simulink library "powerlib_modelsV2"  (Simulink 6.0)
settings: Solver=ode45  SolverMode=SingleTasking  StartTime=0.0  StopTime=10.0  RelTol=1e-3
values from neighbouring files (symbols this model uses):
  Ts = get(handles.edit1,'string')    [powergui.m]
undefined symbols (not defined in the file or in its folder): A, Ac, B, Bc, C, Cc, Cs, Current, damp, Dc, Dd, DiscIntNeverNeededParam, dref, dwo, exc, F, fb, gate, GH, GHd, GI, GId, GL, GLd, H, HT, hyd, ib, ib2, io, isfinite, j, K, Kd, Kg, L, Lad, Laq, lim, LIM, Ll, Llfd, Llkd, Llkq1, Llkq2, Llr, Lls, LowerFlux, N, N2, Nb, Nb2, nb_arm, p, Par_HarmoA_pu, Par_HarmoB_pu, Par_Timing_Harmo, Par_Timing_Variation, Par_Vps, Pb ... (+57)
libraries: powerlib_extras x14
(part 9 of 11)

== system powerlib_modelsV2/Discrete/synchronous_machine/phiq ==
  note: This subsystem computes the quadrature axis flux phiq.
  vq : Inport  Port=1  LatchInput=off
  w : Inport  Port=2  LatchInput=off
  phid : Inport  Port=3  LatchInput=off
  phimq : Inport  Port=4  LatchInput=off
  Discrete-Time Integrator : DiscreteIntegrator  IntegratorMethod=Integration: Trapezoidal  InitialCondition=phiqo  SampleTime=Ts  SaturateOnIntegerOverflow=on  ICPrevOutput=DiscIntNeverNeededParam  ICPrevScaledInput=DiscIntNeverNeededParam
  Product2 : Product  SaturateOnIntegerOverflow=on  InputSameDT=on
  Rs_Ll : Gain  Gain=Rs/Ll  SaturateOnIntegerOverflow=on
  Sum : Sum  Inputs=+-+  SaturateOnIntegerOverflow=on  InputSameDT=on
  Sum6 : Sum  Inputs=+-  SaturateOnIntegerOverflow=on  InputSameDT=on
  Unit Delay1 : UnitDelay  X0=phiqo  SampleTime=Ts
  web_psb : Gain  Gain=web_psb  SaturateOnIntegerOverflow=on
  phiq : Outport  InitialOutput=0
  wires:
  Discrete-Time Integrator/1 -> Unit Delay1/1
  web_psb/1 -> Discrete-Time Integrator/1
  phimq/1 -> Sum6/1
  phid/1 -> Product2/2
  w/1 -> Product2/1
  vq/1 -> Sum/1
  Product2/1 -> Sum/2
  Sum6/1 -> Rs_Ll/1
  Rs_Ll/1 -> Sum/3
  Sum/1 -> web_psb/1
  Unit Delay1/1 -> phiq/1, Sum6/2

== system powerlib_modelsV2/Discrete/synchronous_machine/qd2abc ==
  note: This subsystem converts id,iq to ia,ib,ic.
  sin,cos : Inport  Port=1  LatchInput=off
  iq,id : Inport  Port=2  LatchInput=off
  Fcn : Fcn  Expr=u[3]*u[2] + u[4]*u[1]
  Fcn1 : Fcn  Expr=(u[2]*(-u[3]-sqrt3*u[4]) + u[1]*(sqrt3*u[3]-u[4]))*0.5
  Mux : Mux  Inputs=[ 2 2 ]
  Mux1_ : Mux  Inputs=3
  Sum : Sum  Orientation=down  Inputs=--  SaturateOnIntegerOverflow=on  InputSameDT=on
  ib : Gain  Gain=ib  SaturateOnIntegerOverflow=on
  is(A) : Outport  InitialOutput=0
  is(pu) : Outport  Port=2  InitialOutput=0
  wires:
  ib/1 -> is(A)/1
  Fcn1/1 -> Sum/2, Mux1_/2
  Fcn/1 -> Mux1_/1, Sum/1
  Sum/1 -> Mux1_/3
  Mux1_/1 -> ib/1, is(pu)/1
  Mux/1 -> Fcn/1, Fcn1/1
  sin,cos/1 -> Mux/1
  iq,id/1 -> Mux/2

== system powerlib_modelsV2/Phasors/3_Phase_Prog_Source/Seq A Generation ==
  Enable : Inport  Port=1  LatchInput=off
  Gain3 : Gain  Gain=pi/180  SaturateOnIntegerOverflow=on
  Magnitude-Angle to Complex : MagnitudeAngleToComplex
  Multiport Switch : MultiPortSwitch  Inputs=3  InputSameDT=on
  Negative-sequence : Constant  Value=[0 2*pi/3 -2*pi/3]
  Phase_Harmo : Constant  Value=Phase_Harmo
  Phase_Harmo1 : Constant  Value=Mag_Harmo
  Phase_Harmo2 : Constant  Value=Seq_Harmo
  Positive-sequence : Constant  Value=[0 -2*pi/3 2*pi/3]
  Product1 : Product  SaturateOnIntegerOverflow=on  InputSameDT=on
  Sum : Sum  SaturateOnIntegerOverflow=on  InputSameDT=on
  Sum1 : Sum  SaturateOnIntegerOverflow=on  InputSameDT=on
  Zero-sequence : Constant  Value=[0 0 0]
  valp_nom2 : Constant
  Seq120 : Outport
  wires:
  Enable/1 -> Product1/1
  Phase_Harmo1/1 -> Magnitude-Angle to Complex/1
  Multiport Switch/1 -> Sum/2
  Phase_Harmo/1 -> Gain3/1
  valp_nom2/1 -> Sum1/2
  Phase_Harmo2/1 -> Sum1/1
  Sum1/1 -> Multiport Switch/1
  Product1/1 -> Seq120/1
  Magnitude-Angle to Complex/1 -> Product1/2
  Gain3/1 -> Sum/1
  Negative-sequence/1 -> Multiport Switch/4
  Positive-sequence/1 -> Multiport Switch/3
  Zero-sequence/1 -> Multiport Switch/2
  Sum/1 -> Magnitude-Angle to Complex/2

== system powerlib_modelsV2/Phasors/3_Phase_Prog_Source/Seq B Generation ==
  Enable : Inport  Port=1  LatchInput=off
  Gain3 : Gain  Gain=pi/180  SaturateOnIntegerOverflow=on
  Magnitude-Angle to Complex : MagnitudeAngleToComplex
  Multiport Switch : MultiPortSwitch  Inputs=3  InputSameDT=on
  Negative-sequence : Constant  Value=[0 2*pi/3 -2*pi/3]
  Phase_Harmo : Constant  Value=Phase_Harmo
  Phase_Harmo1 : Constant  Value=Mag_Harmo
  Phase_Harmo2 : Constant  Value=Seq_Harmo
  Positive-sequence : Constant  Value=[0 -2*pi/3 2*pi/3]
  Product1 : Product  SaturateOnIntegerOverflow=on  InputSameDT=on
  Sum : Sum  SaturateOnIntegerOverflow=on  InputSameDT=on
  Sum1 : Sum  SaturateOnIntegerOverflow=on  InputSameDT=on
  Zero-sequence : Constant  Value=[0 0 0]
  valp_nom2 : Constant
  Seq120 : Outport
  wires:
  Sum/1 -> Magnitude-Angle to Complex/2
  Zero-sequence/1 -> Multiport Switch/2
  Positive-sequence/1 -> Multiport Switch/3
  Negative-sequence/1 -> Multiport Switch/4
  Gain3/1 -> Sum/1
  Magnitude-Angle to Complex/1 -> Product1/2
  Product1/1 -> Seq120/1
  Sum1/1 -> Multiport Switch/1
  Phase_Harmo2/1 -> Sum1/1
  valp_nom2/1 -> Sum1/2
  Phase_Harmo/1 -> Gain3/1
  Multiport Switch/1 -> Sum/2
  Phase_Harmo1/1 -> Magnitude-Angle to Complex/1
  Enable/1 -> Product1/1

== system powerlib_modelsV2/Phasors/3_Phase_Prog_Source/Timer ==
  Clock : Clock
  Look-Up Table : Lookup  DialogController=Simulink.DDGSource  InputValues=tv  OutputValues=opv  SaturateOnIntegerOverflow=on
  Out : Outport
  wires:
  Clock/1 -> Look-Up Table/1
  Look-Up Table/1 -> Out/1

== system powerlib_modelsV2/Phasors/3_Phase_Prog_Source/Variation SubSystem ==
  VariationType : Inport  Port=1  LatchInput=off
  Constant : Constant  Value=2
  Constant1 : Constant  Value=0
  Constant2 : Constant
  Constant3 : Constant
  Constant4 : Constant  Value=0
  Constant5 : Constant  Value=0
  Data Type  Conversion1 : DataTypeConversion  SaturateOnIntegerOverflow=on  RndMeth=Zero
  Data Type  Conversion2 : DataTypeConversion  Orientation=up  SaturateOnIntegerOverflow=on  RndMeth=Zero
  Gain1 : Gain  Gain=2*pi  SaturateOnIntegerOverflow=on
  Integrator : Integrator
  Logical Operator : Logic
  Logical Operator1 : Logic  Orientation=up  Operator=NOT
  Memory : Memory  Orientation=left
  Multiport Switch1 : MultiPortSwitch  InputSameDT=on
  Product : Product  SaturateOnIntegerOverflow=on  InputSameDT=on
  Product1 : Product  SaturateOnIntegerOverflow=on  InputSameDT=on
  Product2 : Product  SaturateOnIntegerOverflow=on  InputSameDT=on
  Relational Operator : RelationalOperator  Operator===  InputSameDT=on
  Relational Operator1 : RelationalOperator  Operator===  InputSameDT=on
  Step : Step  Time=Ton_Variation  SampleTime=0
  Step1 : Step  Time=Toff_Variation  Before=1  After=0  SampleTime=0
  Switch{,1..3} (4 alike) : Switch  Threshold=0.5  InputSameDT=on
  Trigonometric Function1 : Trigonometry
  valp_nom6 : Constant  Value=VariationStep
  valp_nom7 : Constant  Value=VariationRate
  valp_nom8 : Constant  Value=VariationMag
  valp_nom9 : Constant  Value=VariationFreq
  Value : Outport
  wires:
  Relational Operator1/1 -> Data Type  Conversion1/1
  Data Type  Conversion2/1 -> Logical Operator1/1
  Trigonometric Function1/1 -> Product/2
  valp_nom8/1 -> Product/1
  valp_nom9/1 -> Gain1/1
  Gain1/1 -> Product1/2
  Product1/1 -> Trigonometric Function1/1
  Product/1 -> Multiport Switch1/4  "Mod"
  valp_nom7/1 -> Switch1/1
  Constant2/1 -> Switch1/3
  Constant4/1 -> Switch/3
  Switch1/1 -> Switch/1
  Constant/1 -> Relational Operator/2
  Switch/1 -> Integrator/1
  Relational Operator/1 -> Switch1/2
  valp_nom6/1 -> Product2/1
  Product2/1 -> Multiport Switch1/2  "Step"
  Integrator/1 -> Product1/1, Multiport Switch1/3  "Ramp"
  VariationType/1 -> Multiport Switch1/1, Relational Operator1/1, Relational Operator/1
  Step/1 -> Switch/2, Product2/2  "Ton"
  Multiport Switch1/1 -> Switch2/1
  Memory/1 -> Switch2/3
  Constant1/1 -> Switch3/1
  Switch2/1 -> Memory/1, Switch3/3
  Switch3/1 -> Value/1
  Constant3/1 -> Relational Operator1/2
  Step1/1 -> Data Type  Conversion2/1, Switch2/2  "Toff"
  Logical Operator/1 -> Switch3/2
  Logical Operator1/1 -> Logical Operator/1
  Constant5/1 -> Multiport Switch1/5
  Data Type  Conversion1/1 -> Logical Operator/2

== system powerlib_modelsV2/Phasors/Dynamic_Load/Break  Alg. Loop I1 ==
  In : Inport  Orientation=left  Port=1  LatchInput=off
  Complex to Real-Imag : ComplexToRealImag  Orientation=left
  Real-Imag to Complex : RealImagToComplex  Orientation=left
  imag : Subsystem  Orientation=left  mask(Transfer Function with Initial Outputs){N=[1], D=[100e-6  1], Y0=imag(I1_init), U0=imag(I1_init)}
      mask prompts: N "Numerator:"; D "Denominator:"; Y0 "Initial output:"; U0 "Initial input:"
      mask help: Vector expressions for numerator, and denominator. Coefficients are in descending powers of s.
      mask init:
      | [A,B,C,Dd]=tf2ss(N,D);if (isempty(Y0));[m,n]=size(A);X0=zeros(1,m); end; if (isempty(U0));[m,p]=size(B);U0=zeros(1,p);end;X0=getxo(A,B,C,Dd,U0,Y0,0);
      mask Help: Specify the initial output for the transfer function.  An optimization routine attempts to determine the appropriate initial states so that the specified initial output is achieved.  For more details, see the m-file getxo.m
      mask Display: dpoly(N,D,'s')
  real : Subsystem  Orientation=left  mask(Transfer Function with Initial Outputs){N=[1], D=[100e-6  1], Y0=real(I1_init), U0=real(I1_init)}
      mask prompts: N "Numerator:"; D "Denominator:"; Y0 "Initial output:"; U0 "Initial input:"
      mask help: Vector expressions for numerator, and denominator. Coefficients are in descending powers of s.
      mask init:
      | [A,B,C,Dd]=tf2ss(N,D);if (isempty(Y0));[m,n]=size(A);X0=zeros(1,m); end; if (isempty(U0));[m,p]=size(B);U0=zeros(1,p);end;X0=getxo(A,B,C,Dd,U0,Y0,0);
      mask Help: Specify the initial output for the transfer function.  An optimization routine attempts to determine the appropriate initial states so that the specified initial output is achieved.  For more details, see the m-file getxo.m
      mask Display: dpoly(N,D,'s')
  Out : Outport  Orientation=left
  wires:
  imag/1(Out1) -> Real-Imag to Complex/2
  Complex to Real-Imag/2 -> imag/1(In1)
  real/1(Out1) -> Real-Imag to Complex/1
  Complex to Real-Imag/1 -> real/1(In1)
  Real-Imag to Complex/1 -> Out/1
  In/1 -> Complex to Real-Imag/1

== system powerlib_modelsV2/Phasors/Dynamic_Load/I1  ==
  note: V2= 1/3(Vab -a*Vbc)
  note: V1= 1/3(Vab -a^2*Vbc)
  note: I1= (S/V1)'
  Vab Vbc cmplx : Inport  Port=1  LatchInput=off
  S=P+jQ : Inport  Port=2  LatchInput=off
  (a^2)/3 : Gain  Gain=1/3*exp(-j*2*pi/3)  SaturateOnIntegerOverflow=on
  Complex to Magnitude-Angle : ComplexToMagnitudeAngle  Output=Magnitude
  Conj1 : Math  Operator=conj  SaturateOnIntegerOverflow=on
  Demux : Demux  Outputs=2
  Gain : Gain  Gain=1/3  SaturateOnIntegerOverflow=on
  Product : Product  Inputs=/*  SaturateOnIntegerOverflow=on  InputSameDT=on
  Sum3 : Sum  Inputs=+-  SaturateOnIntegerOverflow=on  InputSameDT=on
  pu>V : Gain  Orientation=down  Gain=Vnom*sqrt(3)/sqrt(2)  SaturateOnIntegerOverflow=on
  |V1| : Outport
  I1 : Outport  Port=2
  wires:
  (a^2)/3/1 -> Sum3/2
  Demux/2 -> (a^2)/3/1
  Gain/1 -> Sum3/1
  Vab Vbc cmplx/1 -> Demux/1
  Demux/1 -> Gain/1
  Sum3/1 -> Complex to Magnitude-Angle/1, pu>V/1  "V1"
  Complex to Magnitude-Angle/1 -> |V1|/1
  S=P+jQ/1 -> Product/2
  Product/1 -> Conj1/1
  Conj1/1 -> I1/1
  pu>V/1 -> Product/1

== system powerlib_modelsV2/Phasors/Dynamic_Load/Phase currents ==
  note: Ib= a^2*I1
  note: Ia= I1
  I1 : Inport  Port=1  LatchInput=off
  Mux1 : Mux  Inputs=2
  a^2 : Gain  Gain=exp(-j*2*pi/3)  SaturateOnIntegerOverflow=on
  Ia Ib cmplx : Outport
  wires:
  Mux1/1 -> Ia Ib cmplx/1  "ia ib"
  I1/1 -> a^2/1, Mux1/1
  a^2/1 -> Mux1/2

== system powerlib_modelsV2/Phasors/Dynamic_Load/Power ==
  note: V>Vmin :
      |
      |    P=Po*(V/Vo)^np
      |    Q=Qo*(V/Vo)^np
  note: V<Vmin
      | Constant impedance load :
      |
      |  P=Po*kp*V^2
      | Q=Qo*kq*V^2
  note: kp=Vmin^(np-2)/Vo^np
      | kq=Vmin^(nq-2)/Vo^nq
  V1 : Inport  Port=1  LatchInput=off
  Math Function : Math  Operator=square  SaturateOnIntegerOverflow=on
  Mux2 : Mux  Inputs=2
  Mux3 : Mux  Inputs=2
  P0/ (Vo^np) : Gain  Gain=P0/(Mag_V0^np)  SaturateOnIntegerOverflow=on
  Q0/(Vo^nq) : Gain  Gain=Q0/(Mag_V0^nq)  SaturateOnIntegerOverflow=on
  Real-Imag to Complex : RealImagToComplex
  Switch3 : Switch  Threshold=Vmin  InputSameDT=on
  Switch4 : Switch  Threshold=Vmin  InputSameDT=on
  TF_P : Subsystem  mask(Transfer function){T1=Tp1, T2=Tp2, V_Init=P0}
      mask prompts: T1 "Time constant T1 (s):"; T2 "Time constant T2 (s):"; V_Init "Initial input and output :"
      mask help:
      | This block implements a continuous transfer function:
      |
      |          1+T1s
      | H(s)= ------
      |          1+T2s
      |
      | States are initialized according to  initial input and output value so that simulation starts in steady state.
      mask init:
      | numc=[T1 1];
      | denc=[T2 1];
      | [Ac,Bc,Cc,Dc]=tf2ss(numc,denc);
      | 
      | % Compute Initial states
      | I=eye(size(Ac));
      | x0c=inv(-Ac)*Bc*V_Init;
      mask Display: disp('1+T1s\n---\n1+T2s')
  TF_Q : Subsystem  mask(Transfer function){T1=Tq1, T2=Tq2, V_Init=Q0}
      mask prompts: T1 "Time constant T1 (s):"; T2 "Time constant T2 (s):"; V_Init "Initial input and output :"
      mask help:
      | This block implements a continuous transfer function:
      |
      |          1+T1s
      | H(s)= ------
      |          1+T2s
      |
      | States are initialized according to  initial input and output value so that simulation starts in steady state.
      mask init:
      | numc=[T1 1];
      | denc=[T2 1];
      | [Ac,Bc,Cc,Dc]=tf2ss(numc,denc);
      | 
      | % Compute Initial states
      | I=eye(size(Ac));
      | x0c=inv(-Ac)*Bc*V_Init;
      mask Display: disp('1+T1s\n---\n1+T2s')
  V^nq : Fcn  Expr=u[1]^u[2]
  V^nq , : Fcn  Expr=u[1]^u[2]
  Vmin^(np-2) : Gain  Gain=Vmin^(np-2)  SaturateOnIntegerOverflow=on
  Vmin^(nq-2) : Gain  Gain=Vmin^(nq-2)  SaturateOnIntegerOverflow=on
  np : Constant  Value=np
  nq : Constant  Value=nq
  P+jQ : Outport
  wires:
  Switch4/1 -> Q0/(Vo^nq)/1
  Real-Imag to Complex/1 -> P+jQ/1  "S_dyn=  P + j Q"
  P0/ (Vo^np)/1 -> TF_P/1(In1)
  Q0/(Vo^nq)/1 -> TF_Q/1(In1)
  Switch3/1 -> P0/ (Vo^np)/1
  np/1 -> Mux2/2
  Mux2/1 -> V^nq ,/1
  nq/1 -> Mux3/2
  Mux3/1 -> V^nq/1
  V1/1 -> Mux2/1, Mux3/1, Math Function/1, Switch3/2, Switch4/2
  V^nq/1 -> Switch4/1
  Math Function/1 -> Vmin^(np-2)/1, Vmin^(nq-2)/1
  Vmin^(np-2)/1 -> Switch3/3
  V^nq ,/1 -> Switch3/1
  Vmin^(nq-2)/1 -> Switch4/3
  TF_P/1(Out1) -> Real-Imag to Complex/1
  TF_Q/1(Out1) -> Real-Imag to Complex/2

== system powerlib_modelsV2/Phasors/asynchronous_machine/Mechanical ==
  Tm : Inport  Port=1  LatchInput=off
  phiqds1,iqds1 : Inport  Port=2  LatchInput=off
  phiqds2,iqds2 : Inport  Port=3  LatchInput=off
  1\p : Gain  Gain=1/p  SaturateOnIntegerOverflow=on
  1_2H : Gain  Gain=1/(2*H)  SaturateOnIntegerOverflow=on
  1_Tb2 : Gain  Gain=1/Tb2  SaturateOnIntegerOverflow=on
  F : Gain  Orientation=left  Gain=F  SaturateOnIntegerOverflow=on
  Integrator : Integrator  InitialCondition=wmo
  Integrator1 : Integrator  InitialCondition=tho
  Mux4 : Mux  Inputs=3
  Product{1..4} (4 alike) : Product  Inputs=1  SaturateOnIntegerOverflow=on  InputSameDT=on
  Selector : Selector  Elements=[1 4]  InputPortWidth=4
  Selector1 : Selector  Elements=[2 3]  InputPortWidth=4
  Selector2 : Selector  Elements=[1 4]  InputPortWidth=4
  Selector3 : Selector  Elements=[2 3]  InputPortWidth=4
  Sum : Sum  Inputs=-+-  SaturateOnIntegerOverflow=on  InputSameDT=on
  Sum1 : Sum  Inputs=|-+  SaturateOnIntegerOverflow=on  InputSameDT=on
  Sum2 : Sum  Inputs=|-+  SaturateOnIntegerOverflow=on  InputSameDT=on
  Sum3 : Sum  Inputs=|+-  SaturateOnIntegerOverflow=on  InputSameDT=on
  web : Gain  Gain=web  SaturateOnIntegerOverflow=on
  wr,Te,thr : Outport
  wires:
  Selector/1 -> Product1/1
  Selector1/1 -> Product2/1
  phiqds1,iqds1/1 -> Selector1/1, Selector/1
  Product2/1 -> Sum1/2
  Product1/1 -> Sum1/1
  Mux4/1 -> wr,Te,thr/1
  Tm/1 -> 1_Tb2/1
  Sum/1 -> 1_2H/1
  1_2H/1 -> Integrator/1
  Integrator/1 -> F/1, Mux4/1, web/1  "w (pu)"
  F/1 -> Sum/3
  1_Tb2/1 -> Sum/1  "Tm"
  web/1 -> Integrator1/1
  1\p/1 -> Mux4/3
  Integrator1/1 -> 1\p/1
  Selector2/1 -> Product3/1
  Selector3/1 -> Product4/1
  phiqds2,iqds2/1 -> Selector2/1, Selector3/1
  Product4/1 -> Sum2/2
  Product3/1 -> Sum2/1
  Sum1/1 -> Sum3/1  "Pos.seq.Torque"
  Sum3/1 -> Sum/2, Mux4/2
  Sum2/1 -> Sum3/2  "Neg. seq. Torque"

== system powerlib_modelsV2/Phasors/asynchronous_machine/Negative Sequence Model ==
  note: Implementation of
      | V=RI+L.dI/dt  -> dI/dt=-R/L*I  - V
      |
      | In dq components:
      | did/dt= w*(-r/l*id  +iq +vd/l)
      | diq/dt= w*(-r/l*iq -id + vq/l)
      | where r, l, i ,v are in pu
  Vqds2 : Inport  Port=1  LatchInput=off
  s2 : Inport  Port=2  LatchInput=off
  -pi/2  phase shift : Gain  Gain=exp(-j*pi/2)  SaturateOnIntegerOverflow=on
  Complex to Real-Imag : ComplexToRealImag
  Demux : Demux  Outputs=2
  Demux1 : Demux  Outputs=2
  Equivalent R2 L2 : Subsystem
  Gain1 : Gain  Gain=-1  SaturateOnIntegerOverflow=on
  Gain2 : Gain  Orientation=down  Gain=Rs  SaturateOnIntegerOverflow=on
  Gain3 : Gain  Orientation=left  Gain=[1 -1]  SaturateOnIntegerOverflow=on
  Gain4 : Gain  Gain=web  SaturateOnIntegerOverflow=on
  Integrator : Integrator  InitialCondition=[0 0]
  Mux : Mux  Inputs=[1 1 2]
  Product1 : Product  Inputs=**  SaturateOnIntegerOverflow=on  InputSameDT=on
  Product2 : Product  Inputs=*/  SaturateOnIntegerOverflow=on  InputSameDT=on
  Product3 : Product  Inputs=**  SaturateOnIntegerOverflow=on  InputSameDT=on
  Real-Imag to Complex : RealImagToComplex
  Real-Imag to Complex1 : RealImagToComplex
  Selector1 : Selector  Orientation=left  Elements=[2 1]  InputPortWidth=2
  Sum : Sum  Inputs=+-+  SaturateOnIntegerOverflow=on  InputSameDT=on
  Sum1 : Sum  Orientation=down  Inputs=+-  SaturateOnIntegerOverflow=on  InputSameDT=on
  I2s : Outport
  I2r : Outport  Port=2
  Phiqds2_Iqds2 : Outport  Port=3
  wires:
  Real-Imag to Complex1/1 -> I2s/1, Product3/1, Gain2/1
  Demux1/2 -> Real-Imag to Complex1/1
  Demux1/1 -> Real-Imag to Complex1/2
  Gain1/1 -> I2r/1
  Product3/1 -> Gain1/1
  Equivalent R2 L2/3(Zm/(Zr+Zm)) -> Product3/2
  Equivalent R2 L2/1(L2_pu) -> Product2/2
  Product1/1 -> Sum/2  "Iqd2*R2/L2"
  Equivalent R2 L2/2(R2/L2_pu) -> Product1/2
  s2/1 -> Equivalent R2 L2/1(s2)
  Gain4/1 -> Integrator/1
  Sum/1 -> Gain4/1
  Product2/1 -> Sum/1  "Vqd2/L2"
  Integrator/1 -> Demux1/1, Product1/1, Gain3/1, Mux/3  "Iqds2"
  Gain3/1 -> Selector1/1
  Selector1/1 -> Sum/3  "[-id2 iq2]"
  Vqds2/1 -> Product2/1, Demux/1
  Demux/1 -> Real-Imag to Complex/2
  Demux/2 -> Real-Imag to Complex/1
  Gain2/1 -> Sum1/2
  Sum1/1 -> -pi/2  phase shift/1  "Vm2"
  -pi/2  phase shift/1 -> Complex to Real-Imag/1  "Phi2"
  Real-Imag to Complex/1 -> Sum1/1
  Complex to Real-Imag/2 -> Mux/1  "Phiqs2"
  Mux/1 -> Phiqds2_Iqds2/1
  Complex to Real-Imag/1 -> Mux/2  "Phids2"

== system powerlib_modelsV2/Phasors/asynchronous_machine/Positive Sequence Model ==
  Vqdr1 : Inport  Port=1  LatchInput=off
  w-wr : Inport  Port=2  LatchInput=off
  Vqds1 : Inport  Port=3  LatchInput=off
  Constant7 : Constant
  Mutual fluxes : Subsystem  Orientation=left
  Rotor : Subsystem
      mask Display: disp('Rotor')
  Stator : Subsystem
      mask Display: disp('Stator')
  Iqdr1 : Outport
  phiqdr1 : Outport  Port=2
  phiqds1 : Outport  Port=3
  Iqds1 : Outport  Port=4
  Phiqds1_Isqds1 : Outport  Port=5
  wires:
  Stator/3(phis,is) -> Phiqds1_Isqds1/1
  Stator/2(iqs,ids) -> Iqds1/1
  w-wr/1 -> Rotor/2(w-wr)
  Rotor/1(iqr,idr) -> Iqdr1/1
  Vqds1/1 -> Stator/2(vqs,vds)
  Vqdr1/1 -> Rotor/1(vqr,vdr)
  Constant7/1 -> Stator/3(w)
  Rotor/2(phiqr,phidr) -> phiqdr1/1, Mutual fluxes/1(phiqr,phidr)
  Stator/1(phiqs,phids) -> phiqds1/1, Mutual fluxes/2(phiqs,phids)
  Mutual fluxes/1(phimq,phimd) -> Rotor/3(phimq,phimd), Stator/1(phimq,phimd)

== system powerlib_modelsV2/Phasors/asynchronous_machine/abc2dq ==
  note: V2= 1/3(Vab -a*Vbc)
  note: V1= 1/3(Vab -a^2*Vbc)
  Vab Vbc cmplx : Inport  Port=1  LatchInput=off
  (a^2)/3 : Gain  Gain=1/3*exp(-j*2*pi/3)  SaturateOnIntegerOverflow=on
  Complex to Real-Imag : ComplexToRealImag
  Complex to Real-Imag3 : ComplexToRealImag
  Demux : Demux  Outputs=2
  Gain : Gain  Gain=1/3  SaturateOnIntegerOverflow=on
  Gain1 : Gain  Gain=1/3  SaturateOnIntegerOverflow=on
  Mux : Mux  Inputs=2
  Mux3 : Mux  Inputs=2
  Sum3 : Sum  Inputs=+-  SaturateOnIntegerOverflow=on  InputSameDT=on
  Sum4 : Sum  Inputs=+-  SaturateOnIntegerOverflow=on  InputSameDT=on
  a/3 : Gain  Gain=1/3*exp(j*2*pi/3)  SaturateOnIntegerOverflow=on
  Vqds1 : Outport
  Vqds2 : Outport  Port=2
  wires:
  Mux3/1 -> Vqds2/1
  Complex to Real-Imag3/1 -> Mux3/2
  Complex to Real-Imag3/2 -> Mux3/1
  Sum4/1 -> Complex to Real-Imag3/1  "V2"
  (a^2)/3/1 -> Sum3/2
  Demux/2 -> (a^2)/3/1, a/3/1
  Gain/1 -> Sum3/1
  Vab Vbc cmplx/1 -> Demux/1
  Gain1/1 -> Sum4/1
  a/3/1 -> Sum4/2
  Demux/1 -> Gain/1, Gain1/1
  Sum3/1 -> Complex to Real-Imag/1  "V1"
  Complex to Real-Imag/1 -> Mux/2
  Complex to Real-Imag/2 -> Mux/1
  Mux/1 -> Vqds1/1

== system powerlib_modelsV2/Phasors/asynchronous_machine/dq2abc ==
  iqdr1 : Inport  Port=1  LatchInput=off
  iqds1 : Inport  Port=2  LatchInput=off
  Ir2 : Inport  Port=3  LatchInput=off
  Is2 : Inport  Port=4  LatchInput=off
  Phasors Ia Ib rotor : Subsystem
  Phasors Ia Ib stator : Subsystem
  irabc : Outport
  isabc : Outport  Port=2
  wires:
  Is2/1 -> Phasors Ia Ib stator/2(I2s)
  Ir2/1 -> Phasors Ia Ib rotor/2(I2r)
  Phasors Ia Ib rotor/1(Irabc cmplx) -> irabc/1
  Phasors Ia Ib stator/1(Isabc cmplx) -> isabc/1
  iqdr1/1 -> Phasors Ia Ib rotor/1(Iqdr1)
  iqds1/1 -> Phasors Ia Ib stator/1(Iqds1)

== system powerlib_modelsV2/Phasors/simplified_sync_mach/Idq1 Idq2 Pe  ==
  note: I2= -V2/Z
  note: I1= (E-V1)/Z
  note: V1= 1/3(Vab -a^2*Vbc)
  note: V2= 1/3(Vab -a*Vbc)
  Vab Vbc cmplx : Inport  Port=1  LatchInput=off
  e : Inport  Port=2  LatchInput=off
  delta : Inport  Port=3  LatchInput=off
  (a^2)/3 : Gain  Gain=1/3*exp(-j*2*pi/3)  SaturateOnIntegerOverflow=on
  -1 : Gain  Gain=-1  SaturateOnIntegerOverflow=on
  1/Z1 : Gain  Gain=1/(R+j*L)  SaturateOnIntegerOverflow=on
  Complex to Real-Imag : ComplexToRealImag  Output=Real
  Complex to Real-Imag1 : ComplexToRealImag
  Complex to Real-Imag2 : ComplexToRealImag
  Complex to Real-Imag3 : ComplexToRealImag
  Demux : Demux  Outputs=2
  Gain : Gain  Gain=1/3  SaturateOnIntegerOverflow=on
  Gain1 : Gain  Gain=1/3  SaturateOnIntegerOverflow=on
  Magnitude-Angle to Complex1 : MagnitudeAngleToComplex
  Mux1 : Mux  Inputs=2
  Mux2 : Mux  Inputs=2
  Product : Product  SaturateOnIntegerOverflow=on  InputSameDT=on
  Real-Imag to Complex : RealImagToComplex
  Sum1 : Sum  Inputs=-+  SaturateOnIntegerOverflow=on  InputSameDT=on
  Sum3 : Sum  Inputs=+-  SaturateOnIntegerOverflow=on  InputSameDT=on
  Sum4 : Sum  Inputs=+-  SaturateOnIntegerOverflow=on  InputSameDT=on
  Vdq1->Idq1 : Subsystem
  Vdq2->Idq2 : Subsystem
  a/3 : Gain  Gain=1/3*exp(j*2*pi/3)  SaturateOnIntegerOverflow=on
  conj : Gain  Gain=-1  SaturateOnIntegerOverflow=on
  Pe : Outport
  Idq1 : Outport  Port=2
  Idq2 : Outport  Port=3
  wires:
  conj/1 -> Real-Imag to Complex/2
  Complex to Real-Imag1/2 -> conj/1
  Complex to Real-Imag1/1 -> Real-Imag to Complex/1
  Real-Imag to Complex/1 -> Product/2
  Magnitude-Angle to Complex1/1 -> Complex to Real-Imag1/1, Sum1/2  "E"
  Complex to Real-Imag/1 -> Pe/1
  Product/1 -> Complex to Real-Imag/1
  1/Z1/1 -> Product/1
  Sum1/1 -> 1/Z1/1, Complex to Real-Imag2/1  "U1=E1-V1"
  Sum3/1 -> Sum1/1  "V1"
  delta/1 -> Magnitude-Angle to Complex1/2
  e/1 -> Magnitude-Angle to Complex1/1
  Demux/1 -> Gain1/1, Gain/1
  a/3/1 -> Sum4/2
  Gain1/1 -> Sum4/1
  Vab Vbc cmplx/1 -> Demux/1
  Gain/1 -> Sum3/1
  Demux/2 -> a/3/1, (a^2)/3/1
  (a^2)/3/1 -> Sum3/2
  Sum4/1 -> -1/1  "V2"
  -1/1 -> Complex to Real-Imag3/1  "-V2"
  Complex to Real-Imag2/1 -> Mux1/1
  Complex to Real-Imag2/2 -> Mux1/2
  Complex to Real-Imag3/1 -> Mux2/1
  Complex to Real-Imag3/2 -> Mux2/2
  Mux1/1 -> Vdq1->Idq1/1(In1)
  Mux2/1 -> Vdq2->Idq2/1(In1)
  Vdq1->Idq1/1(Out1) -> Idq1/1
  Vdq2->Idq2/1(Out1) -> Idq2/1

== system powerlib_modelsV2/Phasors/simplified_sync_mach/LL2LN ==
  note: Vcn= -Van - Vbn
  note: Vbn=(Vbc - Vab)/3
  note: Van=(2*Vab+Vbc))/3
  Vab_bc : Inport  Port=1  LatchInput=off
  1/3 : Gain  Gain=1/3  SaturateOnIntegerOverflow=on
  2 : Gain  Gain=2  SaturateOnIntegerOverflow=on
  Demux : Demux  Outputs=2
  Mux2 : Mux  Inputs=3
  Sum1 : Sum  SaturateOnIntegerOverflow=on  InputSameDT=on
  Sum2 : Sum  Inputs=+-  SaturateOnIntegerOverflow=on  InputSameDT=on
  Sum6 : Sum  Orientation=down  Inputs=--  SaturateOnIntegerOverflow=on  InputSameDT=on
  Vabc_n : Outport
  wires:
  Demux/2 -> Sum2/1, Sum1/2
  2/1 -> Sum1/1
  Demux/1 -> Sum2/2, 2/1
  1/3/1 -> Demux/1
  Mux2/1 -> Vabc_n/1
  Vab_bc/1 -> 1/3/1
  Sum1/1 -> Sum6/2, Mux2/1  "Van"
  Sum2/1 -> Sum6/1, Mux2/2  "Vbn"
  Sum6/1 -> Mux2/3

== system powerlib_modelsV2/Phasors/simplified_sync_mach/Phasors Ia Ib ==
  note: Ib= a^2*I1 + a*I2
  note: Ia= I1 + I2
  Idq1 : Inport  Port=1  LatchInput=off
  Idq2 : Inport  Port=2  LatchInput=off
  Demux : Demux  Outputs=2
  Demux1 : Demux  Outputs=2
  Mux1 : Mux  Inputs=2
  Mux2 : Mux  Inputs=[2 1]
  Real-Imag to Complex : RealImagToComplex
  Real-Imag to Complex2 : RealImagToComplex
  Sum : Sum  Orientation=down  Inputs=1  SaturateOnIntegerOverflow=on  InputSameDT=on
  Sum1 : Sum  SaturateOnIntegerOverflow=on  InputSameDT=on
  Sum3 : Sum  SaturateOnIntegerOverflow=on  InputSameDT=on
  a : Gain  Gain=exp(j*2*pi/3)  SaturateOnIntegerOverflow=on
  a^2 : Gain  Gain=exp(-j*2*pi/3)  SaturateOnIntegerOverflow=on
  inv : Gain  Gain=-1  SaturateOnIntegerOverflow=on
  Iabc cmplx : Outport
  Iab cmplx : Outport  Port=2
  wires:
  Real-Imag to Complex2/1 -> a/1, Sum3/2  "I2"
  Idq2/1 -> Demux1/1
  Demux1/2 -> Real-Imag to Complex2/2
  Demux1/1 -> Real-Imag to Complex2/1
  Real-Imag to Complex/1 -> Sum3/1, a^2/1  "I1"
  Mux2/1 -> Iabc cmplx/1
  inv/1 -> Mux2/2  "ic"
  Sum/1 -> inv/1
  Mux1/1 -> Sum/1, Mux2/1, Iab cmplx/1  "ia ib"
  Demux/2 -> Real-Imag to Complex/2
  Demux/1 -> Real-Imag to Complex/1
  Idq1/1 -> Demux/1
  Sum1/1 -> Mux1/2
  Sum3/1 -> Mux1/1
  a/1 -> Sum1/2
  a^2/1 -> Sum1/1

== system powerlib_modelsV2/Phasors/simplified_sync_mach/Subsystem ==
  i : Inport  Port=1  LatchInput=off
  v : Inport  Port=2  LatchInput=off
  e : Inport  Port=3  LatchInput=off
  theta : Inport  Port=4  LatchInput=off
  wm : Inport  Port=5  LatchInput=off
  Pe : Inport  Port=6  LatchInput=off
  Gain : Gain  Gain=[ ib2*ones(3,1); Vb3*ones(6,1); 1; Nb; Pb ]  SaturateOnIntegerOverflow=on
  Mux : Mux  Inputs=[ 3 3 3 1 1 1 ]
  * : Outport  InitialOutput=0
  wires:
  Gain/1 -> */1
  Mux/1 -> Gain/1
  Pe/1 -> Mux/6
  wm/1 -> Mux/5
  theta/1 -> Mux/4
  e/1 -> Mux/3
  v/1 -> Mux/2
  i/1 -> Mux/1

== system powerlib_modelsV2/Phasors/simplified_sync_mach/mechanics ==
  Pm : Inport  Port=1  LatchInput=off
  Pe : Inport  Port=2  LatchInput=off
  1_(2*H) : Gain  Gain=1/(2*H)  SaturateOnIntegerOverflow=on
  1_Pb : Gain  Gain=1/Pb  SaturateOnIntegerOverflow=on
  Gain : Gain  Orientation=left  Gain=Kd  SaturateOnIntegerOverflow=on
  Integrator : Integrator  InitialCondition=dwo
  Integrator1 : Integrator  InitialCondition=tho
  Mux1 : Mux  Inputs=2
  Sum : Sum  SaturateOnIntegerOverflow=on  InputSameDT=on
  Sum1 : Sum  Inputs=+-  SaturateOnIntegerOverflow=on  InputSameDT=on
  Sum2 : Sum  Inputs=-+  SaturateOnIntegerOverflow=on  InputSameDT=on
  div : Fcn  Expr=u[2]/u[1]
      mask Display: disp('division')
  nom. speed : Constant
  web : Gain  Gain=web  SaturateOnIntegerOverflow=on
  theta_e : Outport  InitialOutput=0
  wm : Outport  Port=2  InitialOutput=0
  wires:
  Pm/1 -> 1_Pb/1
  1_Pb/1 -> Sum2/2
  web/1 -> Integrator1/1
  Integrator1/1 -> theta_e/1
  Mux1/1 -> div/1
  Pe/1 -> Sum2/1
  Sum2/1 -> Mux1/2
  Sum/1 -> Mux1/1, wm/1, web/1
  1_(2*H)/1 -> Integrator/1
  div/1 -> Sum1/1
  Gain/1 -> Sum1/2
  Sum1/1 -> 1_(2*H)/1
  Integrator/1 -> Sum/2, Gain/1
  nom. speed/1 -> Sum/1

== system powerlib_modelsV2/Phasors/synchronous_machine/Delta angle ==
  Vq : Inport  Port=1  PortDimensions=1  LatchInput=off
  Vd : Inport  Port=2  PortDimensions=1  LatchInput=off
  Cartesian to Polar : Subsystem
      mask Type: Cart2Polar
      mask Description:
      | Transformation from cartesian to polar coordinates.
      | [x, y] -> [r, theta]
      | 
      | r = sqrt(x^2 + y^2);
      | theta = atan(y/x);
      mask Help: Unmask this block for more help.
      mask Display: plot(0,0,100,100,[24,20,15,20,20],[85,95,85,95,20],[80,20,95,85,95,85],[70,20,20,15,20,24],[56,56,55,52,50,46],[20,26,31,35,38,42])
  Radians to Degrees : Subsystem
      mask Type: RadiansToDegrees
      mask Description:
      | Conversion from Radians to Degrees.
      | 
      | D=180/pi*R
      mask Help: This block converts from Radians to Degrees.
      mask Display: disp('R2D')
  Terminator2 : Terminator
  delta : Outport
  wires:
  Vd/1 -> Cartesian to Polar/2(y)
  Radians to Degrees/1(Degrees out) -> delta/1  "delta"
  Vq/1 -> Cartesian to Polar/1(x)
  Cartesian to Polar/1(r) -> Terminator2/1
  Cartesian to Polar/2(theta) -> Radians to Degrees/1(Radians in)

== system powerlib_modelsV2/Phasors/synchronous_machine/PQ ==
  note: P = Vd*Id + Vq*Iq
  note: Q = Vq*Id-Vd*Iq
  note: PQ Measurement:
  Vq : Inport  Port=1  PortDimensions=1  LatchInput=off
  Vd : Inport  Port=2  PortDimensions=1  LatchInput=off
  Iq : Inport  Port=3  PortDimensions=2  LatchInput=off
  Demux1 : Demux  Outputs=[1,1]
  Gain : Gain  Gain=Gain1  SaturateOnIntegerOverflow=on
  Gain1 : Gain  Gain=Gain1  SaturateOnIntegerOverflow=on
  Product{2..5} (4 alike) : Product  SaturateOnIntegerOverflow=on  InputSameDT=on
  Sum : Sum  SaturateOnIntegerOverflow=on  InputSameDT=on
  Sum1 : Sum  Inputs=+-  SaturateOnIntegerOverflow=on  InputSameDT=on
  Peo : Outport
  Qeo : Outport  Port=2
  wires:
  Demux1/1 -> Product5/2, Product2/2
  Iq/1 -> Demux1/1
  Gain1/1 -> Qeo/1
  Gain/1 -> Peo/1
  Product2/1 -> Sum/1
  Product3/1 -> Sum/2
  Product4/1 -> Sum1/1
  Product5/1 -> Sum1/2
  Sum/1 -> Gain/1  "Peo"
  Sum1/1 -> Gain1/1  "Qeo"
  Vd/1 -> Product3/1, Product5/1
  Vq/1 -> Product2/1, Product4/1
  Demux1/2 -> Product3/2, Product4/2

== system powerlib_modelsV2/Phasors/synchronous_machine/Phasors Ia Ib ==
  note: add angle d_theta
  note: Ib= a^2*I1 + a*I2
  note: Ia= I1 + I2
  Idq1 : Inport  Port=1  LatchInput=off
  d_theta : Inport  Port=2  LatchInput=off
  I2_cmplx : Inport  Port=3  LatchInput=off
  Demux : Demux  Outputs=2
  Gain2 : Gain  Gain=j  SaturateOnIntegerOverflow=on
  Math Function : Math  SaturateOnIntegerOverflow=on
  Mux1 : Mux  Inputs=2
  Mux2 : Mux  Inputs=[2 1]
  Product : Product  SaturateOnIntegerOverflow=on  InputSameDT=on
  Real-Imag to Complex : RealImagToComplex
  Sum : Sum  Orientation=down  Inputs=1  SaturateOnIntegerOverflow=on  InputSameDT=on
  Sum1 : Sum  SaturateOnIntegerOverflow=on  InputSameDT=on
  Sum3 : Sum  SaturateOnIntegerOverflow=on  InputSameDT=on
  a : Gain  Gain=exp(j*2*pi/3)  SaturateOnIntegerOverflow=on
  a^2 : Gain  Gain=exp(-j*2*pi/3)  SaturateOnIntegerOverflow=on
  inv : Gain  Gain=-1  SaturateOnIntegerOverflow=on
  Ia Ib cmplx : Outport
  Iabc cmplx : Outport  Port=2
  wires:
  d_theta/1 -> Gain2/1
  Real-Imag to Complex/1 -> Product/1  "I1 machine"
  Math Function/1 -> Product/2
  Gain2/1 -> Math Function/1
  Mux2/1 -> Iabc cmplx/1
  inv/1 -> Mux2/2  "ic"
  Sum/1 -> inv/1
  Mux1/1 -> Mux2/1, Ia Ib cmplx/1, Sum/1  "ia ib"
  Demux/2 -> Real-Imag to Complex/2
  Demux/1 -> Real-Imag to Complex/1
  Idq1/1 -> Demux/1
  Product/1 -> Sum3/1, a^2/1  "I1"
  Sum1/1 -> Mux1/2
  Sum3/1 -> Mux1/1
  a/1 -> Sum1/2
  a^2/1 -> Sum1/1
  I2_cmplx/1 -> Sum3/2, a/1  "I2"

== system powerlib_modelsV2/Phasors/synchronous_machine/Subsystem ==
  Vf : Inport  Port=1  LatchInput=off
  Constant : Constant  Value=excAxis
  Ground2 : Ground
  Switch : Switch  Threshold=1.5  InputSameDT=on
  Switch1 : Switch  Threshold=1.5  InputSameDT=on
  Vkq1 : Outport
  Vfd : Outport  Port=2
  wires:
  Switch/1 -> Vkq1/1
  Switch1/1 -> Vfd/1
  Constant/1 -> Switch1/2, Switch/2
  Vf/1 -> Switch/1, Switch1/3
  Ground2/1 -> Switch/3, Switch1/1

== system powerlib_modelsV2/Phasors/synchronous_machine/Vd1 Vq1, I2  ==
  note: Subtract angle d_theta
  note: I2=-V2/(R2+ j*X2)
      | where X2=2(X''d*X''q/(X"d+X"q) ; R2=X2/30
  note: V2= 1/3(Vab -a*Vbc)
  note: V1= 1/3(Vab -a^2*Vbc)
  Vab Vbc cmplx : Inport  Port=1  LatchInput=off
  d_theta : Inport  Port=2  LatchInput=off
  (a^2)/3 : Gain  Gain=1/3*exp(-j*2*pi/3)  SaturateOnIntegerOverflow=on
  Complex to Real-Imag1 : ComplexToRealImag
  Complex to Real-Imag2 : ComplexToRealImag
  Demux : Demux  Outputs=2
  Gain : Gain  Gain=1/3  SaturateOnIntegerOverflow=on
  Gain1 : Gain  Gain=1/3  SaturateOnIntegerOverflow=on
  Gain2 : Gain  Gain=-j  SaturateOnIntegerOverflow=on
  Math Function : Math  SaturateOnIntegerOverflow=on
  Mux2 : Mux  Inputs=2
  Product : Product  SaturateOnIntegerOverflow=on  InputSameDT=on
  Sum3 : Sum  Inputs=+-  SaturateOnIntegerOverflow=on  InputSameDT=on
  Sum4 : Sum  Inputs=+-  SaturateOnIntegerOverflow=on  InputSameDT=on
  Vdq2->Idq2 : Subsystem
  a/3 : Gain  Gain=1/3*exp(j*2*pi/3)  SaturateOnIntegerOverflow=on
  Vd : Outport
  Vq : Outport  Port=2
  I2_cmplx : Outport  Port=3
  wires:
  Math Function/1 -> Product/2
  Product/1 -> Complex to Real-Imag1/1
  Gain2/1 -> Math Function/1
  Sum4/1 -> Complex to Real-Imag2/1  "V2"
  (a^2)/3/1 -> Sum3/2
  Demux/2 -> (a^2)/3/1, a/3/1
  Complex to Real-Imag1/1 -> Vd/1
  Complex to Real-Imag1/2 -> Vq/1
  Sum3/1 -> Product/1  "V1"
  d_theta/1 -> Gain2/1
  Gain/1 -> Sum3/1
  Vab Vbc cmplx/1 -> Demux/1
  Gain1/1 -> Sum4/1
  a/3/1 -> Sum4/2
  Demux/1 -> Gain/1, Gain1/1
  Complex to Real-Imag2/1 -> Mux2/1
  Complex to Real-Imag2/2 -> Mux2/2
  Mux2/1 -> Vdq2->Idq2/1(V2_dq)
  Vdq2->Idq2/1(I2_cmplx) -> I2_cmplx/1

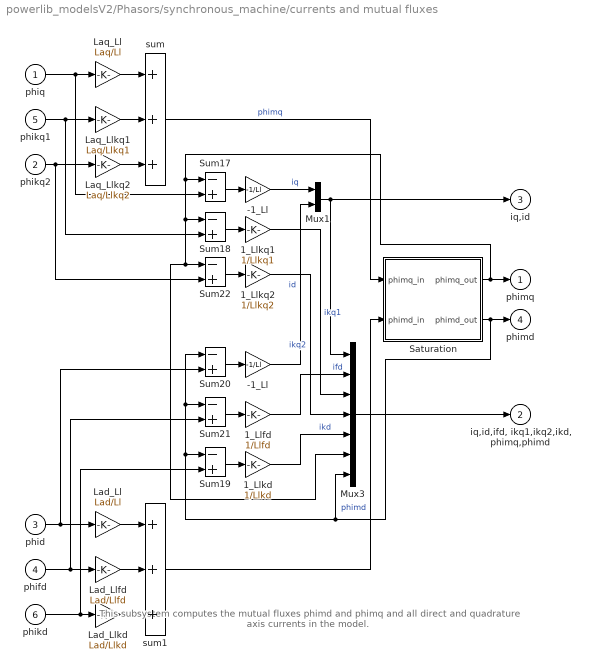
== system powerlib_modelsV2/Phasors/synchronous_machine/currents and mutual fluxes ==
  note: This subsystem computes the mutual fluxes phimd
      | and phimq and all direct and quadrature axis
      | currents in the model.
  phiq : Inport  Port=1  LatchInput=off
  phikq2 : Inport  Port=2  LatchInput=off
  phid : Inport  Port=3  LatchInput=off
  phifd : Inport  Port=4  LatchInput=off
  phikq1 : Inport  Port=5  LatchInput=off
  phikd : Inport  Port=6  LatchInput=off
  -1_Ll : Gain  Gain=-1/Ll  SaturateOnIntegerOverflow=on
  "-1_Ll " : Gain  Gain=-1/Ll  SaturateOnIntegerOverflow=on
  1_Llfd : Gain  Gain=1/Llfd  SaturateOnIntegerOverflow=on
  1_Llkd : Gain  Gain=1/Llkd  SaturateOnIntegerOverflow=on
  1_Llkq1 : Gain  Gain=1/Llkq1  SaturateOnIntegerOverflow=on
  1_Llkq2 : Gain  Gain=1/Llkq2  SaturateOnIntegerOverflow=on
  Lad_Ll : Gain  Gain=Lad/Ll  SaturateOnIntegerOverflow=on
  Lad_Llfd : Gain  Gain=Lad/Llfd  SaturateOnIntegerOverflow=on
  Lad_Llkd : Gain  Gain=Lad/Llkd  SaturateOnIntegerOverflow=on
  Laq_Ll : Gain  Gain=Laq/Ll  SaturateOnIntegerOverflow=on
  Laq_Llkq1 : Gain  Gain=Laq/Llkq1  SaturateOnIntegerOverflow=on
  Laq_Llkq2 : Gain  Gain=Laq/Llkq2  SaturateOnIntegerOverflow=on
  Mux1 : Mux  Inputs=2
  Mux3 : Mux  Inputs=[2 1 1 1 1 1 1]
  Saturation : Subsystem
  Sum{17..22} (6 alike) : Sum  Inputs=-+  SaturateOnIntegerOverflow=on  InputSameDT=on
  sum : Sum  Inputs=+++  SaturateOnIntegerOverflow=on  InputSameDT=on
  sum1 : Sum  Inputs=+++  SaturateOnIntegerOverflow=on  InputSameDT=on
  phimq : Outport  InitialOutput=0
  "iq,id,ifd, ikq1,ikq2,ikd, phimq,phimd" : Outport  Port=2  InitialOutput=0
  iq,id : Outport  Port=3  InitialOutput=0
  phimd : Outport  Port=4  InitialOutput=0
  wires:
  Saturation/2(phimd_out) -> Mux3/7, Sum19/1, Sum21/1, Sum20/1, phimd/1
  Saturation/1(phimq_out) -> Sum17/1, Mux3/6, Sum22/1, Sum18/1, phimq/1
  sum1/1 -> Saturation/2(phimd_in)  "phimd"
  sum/1 -> Saturation/1(phimq_in)  "phimq"
  Mux3/1 -> "iq,id,ifd, ikq1,ikq2,ikd, phimq,phimd"/1
  1_Llkq2/1 -> Mux3/4  "ikq2"
  1_Llkq1/1 -> Mux3/3  "ikq1"
  Sum20/1 -> "-1_Ll "/1
  "-1_Ll "/1 -> Mux1/2  "id"
  Sum21/1 -> 1_Llfd/1
  Sum19/1 -> 1_Llkd/1
  1_Llfd/1 -> Mux3/2  "ifd"
  1_Llkd/1 -> Mux3/5  "ikd"
  Sum18/1 -> 1_Llkq1/1
  Sum17/1 -> -1_Ll/1
  Sum22/1 -> 1_Llkq2/1
  -1_Ll/1 -> Mux1/1  "iq"
  Mux1/1 -> iq,id/1, Mux3/1
  Lad_Llkd/1 -> sum1/3
  Lad_Llfd/1 -> sum1/2
  Lad_Ll/1 -> sum1/1
  phifd/1 -> Lad_Llfd/1, Sum21/2
  phid/1 -> Sum20/2, Lad_Ll/1
  phikd/1 -> Lad_Llkd/1, Sum19/2
  phiq/1 -> Laq_Ll/1, Sum17/2
  Laq_Ll/1 -> sum/1
  Laq_Llkq2/1 -> sum/3
  Laq_Llkq1/1 -> sum/2
  phikq2/1 -> Laq_Llkq2/1, Sum22/2
  phikq1/1 -> Laq_Llkq1/1, Sum18/2

== system powerlib_modelsV2/Phasors/synchronous_machine/mec ==
  note: This subsystem models the mechanical part of the machine.
  "iq,id " : Inport  Port=1  LatchInput=off
  phid : Inport  Port=2  LatchInput=off
  phiq : Inport  Port=3  LatchInput=off
  Pm : Inport  Port=4  LatchInput=off
  1_(2H) : Gain  Gain=1/(2*H)  SaturateOnIntegerOverflow=on
  1_Pb : Gain  Gain=1/Pb  SaturateOnIntegerOverflow=on
  Clock : Clock
      settings: Decimation=10
  F : Gain  Orientation=left  Gain=F  SaturateOnIntegerOverflow=on
  Integrator : Integrator  InitialCondition=dwo
  Integrator2 : Integrator  InitialCondition=tho
  Mux : Mux  Inputs=[ 1 1 2 ]
  Mux1 : Mux  Inputs=2
  Mux2 : Mux
  Product : Product  SaturateOnIntegerOverflow=on  InputSameDT=on
  Sum : Sum  SaturateOnIntegerOverflow=on  InputSameDT=on
  Sum2 : Sum  Inputs=+--  SaturateOnIntegerOverflow=on  InputSameDT=on
  Sum3 : Sum  SaturateOnIntegerOverflow=on  InputSameDT=on
  Te : Fcn  Expr=u[1]*u[3]-u[2]*u[4]
  div : Fcn  Expr=u[2]/u[1]
      mask Display: disp('/')
  nom. speed : Constant
  web1 : Gain  Gain=web  SaturateOnIntegerOverflow=on
  web2 : Gain  Gain=web  SaturateOnIntegerOverflow=on
  misc : Outport  InitialOutput=0
  thetae : Outport  Port=2  InitialOutput=0
  we : Outport  Port=3  InitialOutput=0
  "Te " : Outport  Port=4  InitialOutput=0
  wires:
  Integrator2/1 -> Mux2/1, Sum3/1  "d_theta (rad)"
  web2/1 -> Sum3/2
  Clock/1 -> web2/1
  web1/1 -> Integrator2/1
  Integrator/1 -> web1/1, F/1, Mux2/4, Sum/2  "dw"
  Product/1 -> Mux2/3  "Pe"
  nom. speed/1 -> Sum/1
  1_(2H)/1 -> Integrator/1
  div/1 -> Sum2/1
  phiq/1 -> Mux/2
  phid/1 -> Mux/1
  "iq,id "/1 -> Mux/3
  Te/1 -> Sum2/2, Product/2, "Te "/1
  Mux/1 -> Te/1
  Mux1/1 -> div/1
  Pm/1 -> 1_Pb/1
  1_Pb/1 -> Mux1/2
  F/1 -> Sum2/3
  Sum2/1 -> 1_(2H)/1
  Sum/1 -> Mux2/2, Product/1, we/1, Mux1/1  "n"
  Mux2/1 -> misc/1
  Sum3/1 -> thetae/1

== system powerlib_modelsV2/Phasors/synchronous_machine/phid ==
  note: This subsystem computes the direct axis flux phid.
  w : Inport  Port=1  LatchInput=off
  phiq : Inport  Port=2  LatchInput=off
  vd : Inport  Port=3  LatchInput=off
  phimd : Inport  Port=4  LatchInput=off
  Product1 : Product  SaturateOnIntegerOverflow=on  InputSameDT=on
  Rs_Ll : Gain  Gain=Rs/Ll  SaturateOnIntegerOverflow=on
  Sum2 : Sum  Inputs=+++  SaturateOnIntegerOverflow=on  InputSameDT=on
  Sum9 : Sum  Inputs=+-  SaturateOnIntegerOverflow=on  InputSameDT=on
  int : Integrator  InitialCondition=phido
  web : Gain  Gain=web  SaturateOnIntegerOverflow=on
  phid : Outport  InitialOutput=0
  wires:
  int/1 -> Sum9/2, phid/1
  web/1 -> int/1
  Sum2/1 -> web/1
  Rs_Ll/1 -> Sum2/3
  Sum9/1 -> Rs_Ll/1
  Product1/1 -> Sum2/1
  w/1 -> Product1/1
  phiq/1 -> Product1/2
  vd/1 -> Sum2/2
  phimd/1 -> Sum9/1

== system powerlib_modelsV2/Phasors/synchronous_machine/phifd ==
  note: This subsystem computes the field flux phifd.
  vfd : Inport  Port=1  LatchInput=off
  phimd : Inport  Port=2  LatchInput=off
  N : Gain  Gain=N  SaturateOnIntegerOverflow=on
  Rf_Llfd : Gain  Gain=Rf/Llfd  SaturateOnIntegerOverflow=on
  Sum10 : Sum  Inputs=+-  SaturateOnIntegerOverflow=on  InputSameDT=on
  Sum3 : Sum  SaturateOnIntegerOverflow=on  InputSameDT=on
  int : Integrator  InitialCondition=phifdo
  web : Gain  Gain=web  SaturateOnIntegerOverflow=on
  phifd : Outport  InitialOutput=0
  wires:
  N/1 -> Sum3/1
  vfd/1 -> N/1
  Rf_Llfd/1 -> Sum3/2
  Sum10/1 -> Rf_Llfd/1
  phimd/1 -> Sum10/1
  web/1 -> int/1
  int/1 -> phifd/1, Sum10/2
  Sum3/1 -> web/1

== system powerlib_modelsV2/Phasors/synchronous_machine/phikd ==
  note: This subsystem computes the direct axis damper flux phikd.
  phimd : Inport  Port=1  LatchInput=off
  vkd : Inport  Port=2  LatchInput=off
  Rkd_Llkd : Gain  Gain=Rkd/Llkd  SaturateOnIntegerOverflow=on
  Sum11 : Sum  Inputs=-+  SaturateOnIntegerOverflow=on  InputSameDT=on
  Sum4 : Sum  SaturateOnIntegerOverflow=on  InputSameDT=on
  int : Integrator  InitialCondition=phikdo
  web : Gain  Gain=web  SaturateOnIntegerOverflow=on
  phikd : Outport  InitialOutput=0
  wires:
  Rkd_Llkd/1 -> Sum4/1
  Sum11/1 -> Rkd_Llkd/1
  phimd/1 -> Sum11/2
  vkd/1 -> Sum4/2
  web/1 -> int/1
  int/1 -> phikd/1, Sum11/1
  Sum4/1 -> web/1

== system powerlib_modelsV2/Phasors/synchronous_machine/phikq1 ==
  note: This subsystem computes the quadrature axis damper flux phikq.
  phimq : Inport  Port=1  LatchInput=off
  vkq1 : Inport  Port=2  LatchInput=off
  Rkq1_Llkq1 : Gain  Gain=Rkq1/Llkq1  SaturateOnIntegerOverflow=on
  Sum1 : Sum  SaturateOnIntegerOverflow=on  InputSameDT=on
  Sum7 : Sum  Inputs=-+  SaturateOnIntegerOverflow=on  InputSameDT=on
  int : Integrator  InitialCondition=phikq1o
  web : Gain  Gain=web  SaturateOnIntegerOverflow=on
  phikq1 : Outport  InitialOutput=0
  wires:
  int/1 -> Sum7/1, phikq1/1
  web/1 -> int/1
  vkq1/1 -> Sum1/2
  phimq/1 -> Sum7/2
  Sum1/1 -> web/1
  Sum7/1 -> Rkq1_Llkq1/1
  Rkq1_Llkq1/1 -> Sum1/1

== system powerlib_modelsV2/Phasors/synchronous_machine/phikq2 ==
  note: This subsystem computes the quadrature axis damper flux phikq2.
  vkq2 : Inport  Port=1  LatchInput=off
  phimq : Inport  Port=2  LatchInput=off
  Enabled integrator : Subsystem  TreatAsAtomicUnit=on
      mask Display: disp('1/s')
  Rkq2_Llkq2 : Gain  Gain=Rkq2/Llkq2  SaturateOnIntegerOverflow=on
  Sum1 : Sum  SaturateOnIntegerOverflow=on  InputSameDT=on
  Sum7 : Sum  Inputs=-+  SaturateOnIntegerOverflow=on  InputSameDT=on
  web : Gain  Gain=web  SaturateOnIntegerOverflow=on
  wref : Constant  Value=isfinite(Llkq2)
  phikq2 : Outport  InitialOutput=0
  wires:
  wref/1 -> Enabled integrator/Enable
  Enabled integrator/1(Out1) -> phikq2/1, Sum7/1
  web/1 -> Enabled integrator/1(In1)
  Sum7/1 -> Rkq2_Llkq2/1
  vkq2/1 -> Sum1/2
  Rkq2_Llkq2/1 -> Sum1/1
  Sum1/1 -> web/1
  phimq/1 -> Sum7/2

== system powerlib_modelsV2/Phasors/synchronous_machine/phiq ==
  note: This subsystem computes the quadrature axis flux phiq.
  vq : Inport  Port=1  LatchInput=off
  w : Inport  Port=2  LatchInput=off
  phid : Inport  Port=3  LatchInput=off
  phimq : Inport  Port=4  LatchInput=off
  Product2 : Product  SaturateOnIntegerOverflow=on  InputSameDT=on
  Rs_Ll : Gain  Gain=Rs/Ll  SaturateOnIntegerOverflow=on
  Sum : Sum  Inputs=+-+  SaturateOnIntegerOverflow=on  InputSameDT=on
  Sum6 : Sum  Inputs=+-  SaturateOnIntegerOverflow=on  InputSameDT=on
  int1 : Integrator  InitialCondition=phiqo
  web : Gain  Gain=web  SaturateOnIntegerOverflow=on
  phiq : Outport  InitialOutput=0
  wires:
  int1/1 -> Sum6/2, phiq/1
  web/1 -> int1/1
  phimq/1 -> Sum6/1
  phid/1 -> Product2/2
  w/1 -> Product2/1
  vq/1 -> Sum/1
  Product2/1 -> Sum/2
  Sum6/1 -> Rs_Ll/1
  Rs_Ll/1 -> Sum/3
  Sum/1 -> web/1

== system powerlib_modelsV2/Switch Current Source/IGBT/Conduction Logic ==
  iak : Inport  Port=1  LatchInput=off
  Vak : Inport  Port=2  LatchInput=off
  g : Inport  Port=3  LatchInput=off
  " " : RelationalOperator  Operator=>  InputSameDT=on
  "    " : Constant  Value=eps
  "      " : Constant  Value=0
  ". " : Logic
  . 1 : Logic  Operator=OR
  Break Alg. Loop : Subsystem  mask{Nsw=length(Ron)}
      mask prompts: Nsw "number of switches"
  Data Type  Conversion{,1..6} (7 alike) : DataTypeConversion  SaturateOnIntegerOverflow=on  RndMeth=Zero
  I>0 : Relay  OnSwitchValue=1000*eps  OffSwitchValue=0
  I>1.5 : Relay  OnSwitchValue=1.5  OffSwitchValue=0
  Test2 : Switch  Threshold=eps  InputSameDT=on
  Vf : Constant  Value=Vf
  b : RelationalOperator  Operator=>  InputSameDT=on
  n1 : Sum  SaturateOnIntegerOverflow=on  InputSameDT=on
  status : Outport  InitialOutput=0
  wires:
  Data Type  Conversion5/1 -> ". "/2, Test2/2
  Vak/1 -> b/1
  b/1 -> Data Type  Conversion6/1
  " "/1 -> Data Type  Conversion5/1
  Data Type  Conversion6/1 -> ". "/1
  g/1 -> Data Type  Conversion4/1
  Test2/1 -> status/1
  "      "/1 -> Test2/3  "zero current"
  Vf/1 -> b/2
  I>0/1 -> n1/1
  iak/1 -> I>0/1
  n1/1 -> I>1.5/1
  Data Type  Conversion/1 -> n1/2
  . 1/1 -> Data Type  Conversion1/1
  Data Type  Conversion1/1 -> Test2/1
  I>1.5/1 -> Data Type  Conversion2/1
  Data Type  Conversion2/1 -> . 1/1
  Data Type  Conversion3/1 -> . 1/2
  ". "/1 -> Break Alg. Loop/1(In1)
  Break Alg. Loop/1(Out1) -> Data Type  Conversion3/1, Data Type  Conversion/1
  Data Type  Conversion4/1 -> " "/1
  "    "/1 -> " "/2

== system powerlib_modelsV2/Switch Current Source/IGBT/Tail ==
  iak : Inport  Port=1  LatchInput=off
  switch : Inport  Port=2  LatchInput=off
  1 : Constant
  Integrator : Integrator  ExternalReset=falling  LimitOutput=on
  Look-Up  Table : Lookup  DialogController=Simulink.DDGSource  InputValues="[  0   Tf+eps Tf+Tt+2*eps  Tf+Tt+3*eps]"  OutputValues="[  1   0.1*(Tt>0) 0 0]"  SaturateOnIntegerOverflow=on
  Product : Product  SaturateOnIntegerOverflow=on  InputSameDT=on
  Switch : Switch  Threshold=eps  InputSameDT=on
  Iak : Outport  InitialOutput=0
  wires:
  Product/1 -> Switch/3
  Switch/1 -> Iak/1
  Integrator/1 -> Look-Up  Table/1
  1/1 -> Integrator/1
  switch/1 -> Integrator/2, Switch/2
  Look-Up  Table/1 -> Product/2
  iak/1 -> Switch/1, Product/1

== system powerlib_modelsV2/Switch Current Source/detailed_thyristor/Conduction logic ==
  Iak_meas. : Inport  Port=1  LatchInput=off
  Vak : Inport  Port=2  LatchInput=off
  G : Inport  Port=3  LatchInput=off
  "    " : Sum  Inputs=+++-  SaturateOnIntegerOverflow=on  InputSameDT=on
  ". " : Logic
  "0   " : Constant  Value=eps
  0.1 : Constant  Value=0.1
  Break Alg. Loop : Subsystem  mask{Nsw=length(Lon), IC=IC}
      mask prompts: Nsw "number of switches"; IC "initial conditions"
  Data Type  Conversion{1,3,5..6} (4 alike) : DataTypeConversion  SaturateOnIntegerOverflow=on  RndMeth=Zero
  I>1.5 : Relay  OnSwitchValue=1.5  OffSwitchValue=0
  Iak>IL : Relay  OnSwitchValue=eps+IL  OffSwitchValue=0
  Time recovery : Subsystem
  Vak>Vf : Subsystem
  b1 : RelationalOperator  Operator=>  InputSameDT=on
  n1 : Sum  SaturateOnIntegerOverflow=on  InputSameDT=on
  reset : Outport  InitialOutput=0
  wires:
  "0   "/1 -> b1/2
  Data Type  Conversion6/1 -> ". "/2
  b1/1 -> Data Type  Conversion6/1
  Data Type  Conversion5/1 -> ". "/1, Time recovery/2("Vak>Vf ")
  Vak>Vf/1(Vak>Vf) -> Data Type  Conversion5/1
  Data Type  Conversion3/1 -> b1/1
  G/1 -> Data Type  Conversion3/1
  Vak/1 -> Vak>Vf/1(Vak)
  Time recovery/1("TQ ") -> "    "/2
  0.1/1 -> "    "/4
  Iak_meas./1 -> Iak>IL/1
  Iak>IL/1 -> Time recovery/3(Iak>il), n1/1
  n1/1 -> I>1.5/1
  I>1.5/1 -> Time recovery/1(Iak>0), "    "/1
  "    "/1 -> Break Alg. Loop/1(In1)
  ". "/1 -> Data Type  Conversion1/1
  Data Type  Conversion1/1 -> "    "/3, n1/2
  Break Alg. Loop/1(Out1) -> reset/1

== system powerlib_modelsV2/Switch Current Source/detailed_thyristor/Switch-Ron-Lon ==
  Vak : Inport  Port=1  LatchInput=off
  Reset : Inport  Port=2  LatchInput=off
  "0 " : Constant  Orientation=left  Value=0
  "0   " : Constant  Orientation=left  Value=0
  Integrator : Integrator  ExternalReset=rising  InitialConditionSource=external
  L_device : Gain  Gain=1./Lon  SaturateOnIntegerOverflow=on
  R_device : Gain  Orientation=left  Gain=Ron  SaturateOnIntegerOverflow=on
  Step : Step  Orientation=left  Time=eps  Before=IC  After=0  SampleTime=0
  Test : Switch  Threshold=eps  InputSameDT=on
  Vak-Vf-Ron*Iak : Sum  Inputs=-+-  SaturateOnIntegerOverflow=on  InputSameDT=on
  Vf : Constant  Value=Vf
  test : Switch  Threshold=eps  InputSameDT=on
  "Iak  " : Outport  InitialOutput=0
  wires:
  "0 "/1 -> Test/3
  "0   "/1 -> test/3
  Step/1 -> Integrator/3
  Integrator/1 -> Test/1, R_device/1
  L_device/1 -> test/1
  test/1 -> Integrator/1
  Test/1 -> "Iak  "/1
  Vf/1 -> Vak-Vf-Ron*Iak/1
  Vak-Vf-Ron*Iak/1 -> L_device/1
  R_device/1 -> Vak-Vf-Ron*Iak/3
  Vak/1 -> Vak-Vf-Ron*Iak/2
  Reset/1 -> test/2, Integrator/2, Test/2

== system powerlib_modelsV2/Switch Current Source/diode/Conduction logic ==
  Iak : Inport  Port=1  LatchInput=off
  Vak : Inport  Port=2  LatchInput=off
  0 2 : Constant  Value=Vf
  0 3 : Constant  Value=0
  0 4 : Constant  Value=0
  Break Alg. Loop : Subsystem  AncestorBlock=powerlib_models/Switch Current Source/diode/Conduction logic/BAL-PB1  mask{Nsw=length(Lon), IC=IC}
      mask prompts: Nsw "number of switches"; IC "Initial condition"
  Data Type  Conversion1 : DataTypeConversion  SaturateOnIntegerOverflow=on  RndMeth=Zero
  Data Type  Conversion2 : DataTypeConversion  SaturateOnIntegerOverflow=on  RndMeth=Zero
  Data Type  Conversion3 : DataTypeConversion  SaturateOnIntegerOverflow=on  RndMeth=Zero
  b5 : RelationalOperator  Operator=>  InputSameDT=on
  b6 : RelationalOperator  Operator=>  InputSameDT=on
  b7 : RelationalOperator  Operator===  InputSameDT=on
  or2 : Logic  Operator=OR
  or3 : Logic
  status : Outport  InitialOutput=0
  wires:
  Vak/1 -> b6/1  "Vak diode"
  0 3/1 -> b7/2
  0 2/1 -> b6/2
  b6/1 -> Data Type  Conversion2/1  "Voltage > 0"
  or3/1 -> or2/2
  or2/1 -> Break Alg. Loop/1(In1)
  0 4/1 -> b5/2
  b5/1 -> Data Type  Conversion1/1  "Current > 0"
  b7/1 -> Data Type  Conversion3/1  "Current = 0"
  Iak/1 -> b5/1, b7/1  "Iak diode"
  Break Alg. Loop/1(Out1) -> status/1
  Data Type  Conversion1/1 -> or2/1
  Data Type  Conversion2/1 -> or3/1
  Data Type  Conversion3/1 -> or3/2
